simulink model "frenagem_real"  (R2016a)
settings: Solver=ode45  StartTime=0.0  StopTime=200  FixedStep=.03  MaxStep=.1  RelTol=1e-3
libraries: canmsglib x4
settings Model: Creator=vmaraccini  LastModifiedBy=vmaraccini-personal
settings DataIOCC: LimitDataPoints=on  SaveFormat=Array
settings HardwareCC: ProdBitPerPointer=32  ProdLargestAtomicFloat=None  ProdIntDivRoundTo=Undefined  ProdEndianess=Unspecified  ProdWordSize=32  ProdHWDeviceType=32-bit Generic
settings ModelReferenceCC: PropagateSignalLabelsOutOfModel=off
settings ConfigComp: CovModelRefEnable=Off

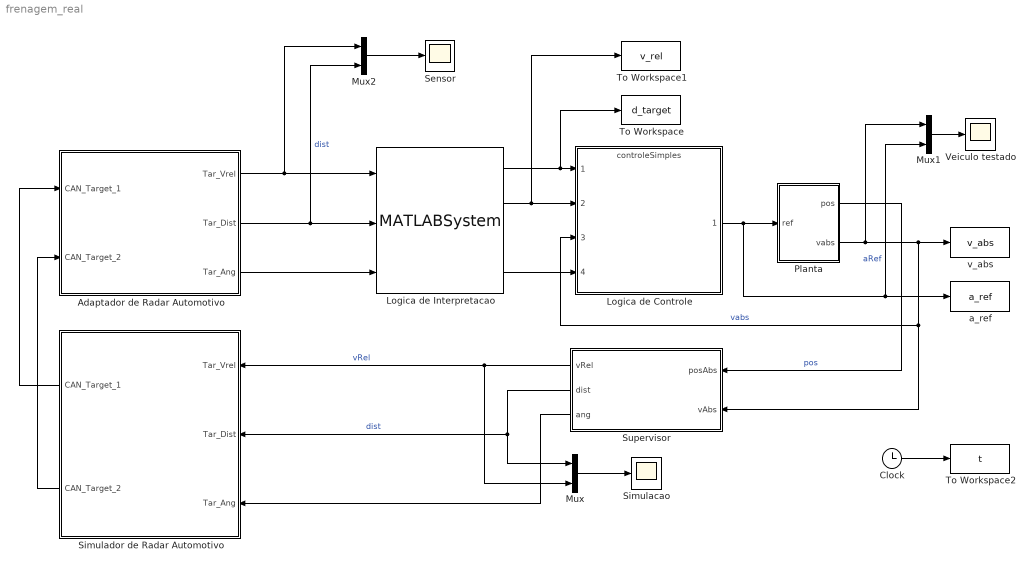
== system frenagem_real ==
  Adaptador de Radar Automotivo : Subsystem
  Clock : Clock
  Logica de Controle : ModelReference  ModelNameDialog=controleSimples.slx  SimulationMode=Normal  ModelReferenceVersion=1.103
  Logica de Interpretacao : MATLABSystem  System=Interpretacao  SimulateUsing=Interpreted execution
      mask Type: Interpretacao
      mask Display:
      | disp('Interpretacao');
      | port_label('input',1,'vrels');
      | port_label('input',2,'dists');
      | port_label('input',3,'angs');
      | port_label('output',1,'dist');
      | port_label('output',2,'vrel');
      | port_label('output',3,'ang');
      | port_label('output',4,'vmax');
  Mux : Mux  Inputs=2
  Mux1 : Mux  Inputs=2
  Mux2 : Mux  Inputs=2
  Planta : Subsystem
  Sensor : Scope
  Simulacao : Scope
  Simulador de Radar Automotivo : Subsystem
  Supervisor : Subsystem
  To Workspace : ToWorkspace  VariableName=d_target  SampleTime=-1
      settings: Save2DSignal=2-D array (concatenate along first dimension)
  To Workspace1 : ToWorkspace  VariableName=v_rel  SampleTime=-1
      settings: Save2DSignal=2-D array (concatenate along first dimension)
  To Workspace2 : ToWorkspace  VariableName=t  SampleTime=-1
      settings: Save2DSignal=2-D array (concatenate along first dimension)
  Veiculo testado : Scope
  a_ref : ToWorkspace  VariableName=a_ref  SampleTime=-1
      settings: Save2DSignal=2-D array (concatenate along first dimension)
  v_abs : ToWorkspace  VariableName=v_abs  SampleTime=-1
      settings: Save2DSignal=2-D array (concatenate along first dimension)
  wires:
  Planta/2(vabs) -> Supervisor/2(vAbs), Logica de Controle/3, v_abs/1, Mux1/1  "vabs"
  Logica de Controle/1 -> Planta/1(ref), Mux1/2, a_ref/1  "aRef"
  Planta/1(pos) -> Supervisor/1(posAbs)  "pos"
  Simulador de Radar Automotivo/1(CAN_Target_1) -> Adaptador de Radar Automotivo/1(CAN_Target_1)
  Simulador de Radar Automotivo/2(CAN_Target_2) -> Adaptador de Radar Automotivo/2(CAN_Target_2)
  Logica de Interpretacao/1 -> To Workspace/1, Logica de Controle/1
  Supervisor/1(vRel) -> Simulador de Radar Automotivo/1(Tar_Vrel), Mux/2  "vRel"
  Supervisor/2(dist) -> Simulador de Radar Automotivo/2(Tar_Dist), Mux/1  "dist"
  Mux/1 -> Simulacao/1
  Mux1/1 -> Veiculo testado/1
  Logica de Interpretacao/4 -> Logica de Controle/4
  Logica de Interpretacao/2 -> Logica de Controle/2, To Workspace1/1
  Supervisor/3(ang) -> Simulador de Radar Automotivo/3(Tar_Ang)
  Adaptador de Radar Automotivo/3(Tar_Ang) -> Logica de Interpretacao/3
  Adaptador de Radar Automotivo/1(Tar_Vrel) -> Mux2/1, Logica de Interpretacao/1
  Adaptador de Radar Automotivo/2(Tar_Dist) -> Mux2/2, Logica de Interpretacao/2  "dist"
  Mux2/1 -> Sensor/1
  Clock/1 -> To Workspace2/1

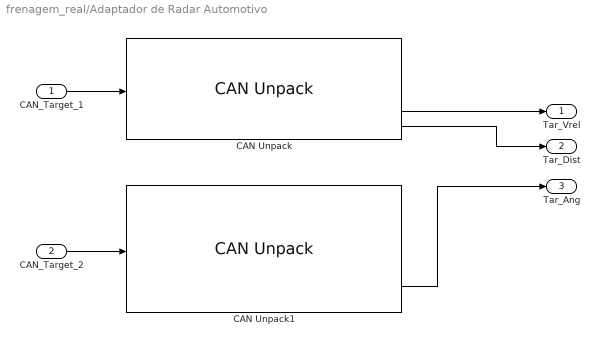
== system frenagem_real/Adaptador de Radar Automotivo ==
  CAN_Target_1 : Inport
  CAN_Target_2 : Inport  Port=2
  CAN Unpack : canmsglib/CAN Unpack  MsgList=(none)  MsgName=CAN1_Target_1  MsgIDType=Standard (11-bit identifier)  MsgIdentifier=1793  MsgLength=8  SignalInfo=NoOfTarget_1$0$8$2$2$1$0$1$0$-Inf$Inf$#Tar_Dist_rms$8$8$2$2$1$0$0.1$-10$-Inf$Inf$#Tar_Ang_rms$17$7$2$2$1$0$0.1$0$-Inf$Inf$#Tar_Vrel_rms$24$9$2$2$1$0$0.03$-5$-Inf$Inf$#Tar_Vrel$44$12$2$2$1$0$0.03$-25$-Inf$Inf$#Tar_Dist$48$11$2$1$1$0$0.1$0$-Inf$Inf$#  NSignals=6  IDPort=off  TimestampPort=off  ErrorPort=off  RemotePort=off  LengthPort=off  StatusPort=off  StartBits=str2num('[int32(0);int32(8);int32(17);int32(24);int32(44);int32(48)]')  SignalSizes=str2num('[int32(8);int32(8);int32(7);int32(9);int32(12);int32(11)]')  ByteOrders=str2num('[int32(2);int32(2);int32(2);int32(2);int32(2);int32(2)]')  DataTypes=str2num('[int32(2);int32(2);int32(2);int32(2);int32(2);int32(1)]')  MultiplexTypes=str2num('[int32(1);int32(1);int32(1);int32(1);int32(1);int32(1)]')  MultiplexValues=str2num('[double(0);double(0);double(0);double(0);double(0);double(0)]')  Factors=str2num('[double(1);double(0.1);double(0.1);double(0.03);double(0.03);double(0.1)]')  Offsets=str2num('[double(0);double(-10);double(0);double(-5);double(-25);double(0)]')  Minimums=str2num('[double(-Inf);double(-Inf);double(-Inf);double(-Inf);double(-Inf);double(-Inf)]')  Maximums=str2num('[double(Inf);double(Inf);double(Inf);double(Inf);double(Inf);double(Inf)]')
  CAN Unpack1 : canmsglib/CAN Unpack  MsgList=(none)  MsgName=CAN1_Target_2  MsgIDType=Standard (11-bit identifier)  MsgIdentifier=1794  MsgLength=8  SignalInfo=NoOfTarget_2$0$8$2$2$1$0$1$0$-Inf$Inf$#Tar_PdH0$9$7$2$2$1$0$0.01$0$-Inf$Inf$#Tar_Length$16$9$2$2$1$0$0.1$0$-Inf$Inf$#Tar_Width$32$9$2$2$1$0$0.1$0$-Inf$Inf$#Tar_Ang_stat$44$2$2$2$1$0$1$0$-Inf$Inf$#Tar_Type$46$2$2$2$1$0$1$0$-Inf$Inf$#Tar_Ang$50$10$2$2$1$0$0.1$-30$-Inf$Inf$#Tar_RCSValue$56$10$2$2$1$0$0.1$-50$-Inf$Inf$#  NSignals=8  IDPort=off  TimestampPort=off  ErrorPort=off  RemotePort=off  LengthPort=off  StatusPort=off  StartBits=str2num('[int32(0);int32(9);int32(16);int32(32);int32(44);int32(46);int32(50);int32(56)]')  SignalSizes=str2num('[int32(8);int32(7);int32(9);int32(9);int32(2);int32(2);int32(10);int32(10)]')  ByteOrders=str2num('[int32(2);int32(2);int32(2);int32(2);int32(2);int32(2);int32(2);int32(2)]')  DataTypes=str2num('[int32(2);int32(2);int32(2);int32(2);int32(2);int32(2);int32(2);int32(2)]')  MultiplexTypes=str2num('[int32(1);int32(1);int32(1);int32(1);int32(1);int32(1);int32(1);int32(1)]')  MultiplexValues=str2num('[double(0);double(0);double(0);double(0);double(0);double(0);double(0);double(0)]')  Factors=str2num('[double(1);double(0.01);double(0.1);double(0.1);double(1);double(1);double(0.1);double(0.1)]')  Offsets=str2num('[double(0);double(0);double(0);double(0);double(0);double(0);double(-30);double(-50)]')  Minimums=str2num('[double(-Inf);double(-Inf);double(-Inf);double(-Inf);double(-Inf);double(-Inf);double(-Inf);double(-Inf)]')  Maximums=str2num('[double(Inf);double(Inf);double(Inf);double(Inf);double(Inf);double(Inf);double(Inf);double(Inf)]')
  Tar_Vrel : Outport
  Tar_Dist : Outport  Port=2
  Tar_Ang : Outport  Port=3
  wires:
  CAN Unpack/6 -> Tar_Dist/1
  CAN Unpack1/7 -> Tar_Ang/1
  CAN Unpack/5 -> Tar_Vrel/1
  CAN_Target_2/1 -> CAN Unpack1/1
  CAN_Target_1/1 -> CAN Unpack/1

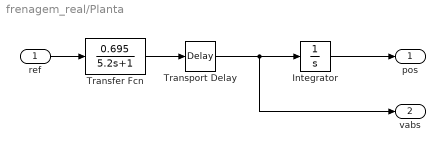
== system frenagem_real/Planta ==
  ref : Inport
  Integrator : Integrator
  Transfer Fcn : TransferFcn  Numerator=[0 0.695]  Denominator=[5.2 1]
  Transport Delay : TransportDelay  DelayTime=0.5
  pos : Outport
  vabs : Outport  Port=2
  wires:
  Integrator/1 -> pos/1
  Transfer Fcn/1 -> Transport Delay/1
  ref/1 -> Transfer Fcn/1
  Transport Delay/1 -> vabs/1, Integrator/1

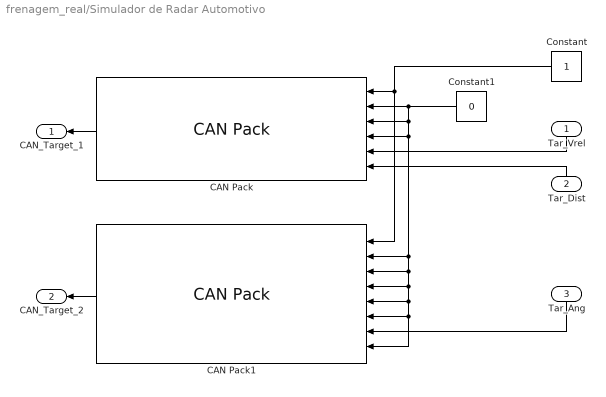
== system frenagem_real/Simulador de Radar Automotivo ==
  Tar_Vrel : Inport
  Tar_Dist : Inport  Port=2
  Tar_Ang : Inport  Port=3
  CAN Pack : canmsglib/CAN Pack  MsgList=(none)  MsgName=CAN1_Target_1  MsgIDType=Standard (11-bit identifier)  MsgIdentifier=1793  MsgLength=8  SignalInfo=NoOfTarget_1$0$8$2$2$1$0$1$0$-Inf$Inf$#Tar_Dist_rms$8$8$2$2$1$0$0.1$-10$-Inf$Inf$#Tar_Ang_rms$17$7$2$2$1$0$0.1$0$-Inf$Inf$#Tar_Vrel_rms$24$9$2$2$1$0$0.03$-5$-Inf$Inf$#Tar_Vrel$44$12$2$2$1$0$0.03$-25$-Inf$Inf$#Tar_Dist$48$11$2$2$1$0$0.1$0$-Inf$Inf$#  NSignals=6  StartBits=str2num('[int32(0);int32(8);int32(17);int32(24);int32(44);int32(48)]')  SignalSizes=str2num('[int32(8);int32(8);int32(7);int32(9);int32(12);int32(11)]')  ByteOrders=str2num('[int32(2);int32(2);int32(2);int32(2);int32(2);int32(2)]')  DataTypes=str2num('[int32(2);int32(2);int32(2);int32(2);int32(2);int32(2)]')  MultiplexTypes=str2num('[int32(1);int32(1);int32(1);int32(1);int32(1);int32(1)]')  MultiplexValues=str2num('[double(0);double(0);double(0);double(0);double(0);double(0)]')  Factors=str2num('[double(1);double(0.1);double(0.1);double(0.03);double(0.03);double(0.1)]')  Offsets=str2num('[double(0);double(-10);double(0);double(-5);double(-25);double(0)]')  Minimums=str2num('[double(-Inf);double(-Inf);double(-Inf);double(-Inf);double(-Inf);double(-Inf)]')  Maximums=str2num('[double(Inf);double(Inf);double(Inf);double(Inf);double(Inf);double(Inf)]')  Remote=off
      settings: DataFormat=manually specified signals
  CAN Pack1 : canmsglib/CAN Pack  MsgList=(none)  MsgName=CAN1_Target_2  MsgIDType=Standard (11-bit identifier)  MsgIdentifier=1794  MsgLength=8  SignalInfo=NoOfTarget_2$0$8$2$2$1$0$1$0$-Inf$Inf$#Tar_PdH0$9$7$2$2$1$0$0.01$-10$-Inf$Inf$#Tar_Length$16$9$2$2$1$0$0.1$0$-Inf$Inf$#Tar_Width$32$9$2$2$1$0$.01$0$-Inf$Inf$#Tar_Ang_stat$44$2$2$2$1$0$1$0$-Inf$Inf$#Tar_Type$46$2$2$2$1$0$1$0$-Inf$Inf$#Tar_Ang$50$10$2$2$1$0$0.1$-30$-Inf$Inf$#Tar_RCSValue$56$10$2$2$1$0$0.1$-50$-Inf$Inf$#  NSignals=8  StartBits=str2num('[int32(0);int32(9);int32(16);int32(32);int32(44);int32(46);int32(50);int32(56)]')  SignalSizes=str2num('[int32(8);int32(7);int32(9);int32(9);int32(2);int32(2);int32(10);int32(10)]')  ByteOrders=str2num('[int32(2);int32(2);int32(2);int32(2);int32(2);int32(2);int32(2);int32(2)]')  DataTypes=str2num('[int32(2);int32(2);int32(2);int32(2);int32(2);int32(2);int32(2);int32(2)]')  MultiplexTypes=str2num('[int32(1);int32(1);int32(1);int32(1);int32(1);int32(1);int32(1);int32(1)]')  MultiplexValues=str2num('[double(0);double(0);double(0);double(0);double(0);double(0);double(0);double(0)]')  Factors=str2num('[double(1);double(0.01);double(0.1);double(.01);double(1);double(1);double(0.1);double(0.1)]')  Offsets=str2num('[double(0);double(-10);double(0);double(0);double(0);double(0);double(-30);double(-50)]')  Minimums=str2num('[double(-Inf);double(-Inf);double(-Inf);double(-Inf);double(-Inf);double(-Inf);double(-Inf);double(-Inf)]')  Maximums=str2num('[double(Inf);double(Inf);double(Inf);double(Inf);double(Inf);double(Inf);double(Inf);double(Inf)]')  Remote=off
      settings: DataFormat=manually specified signals
  Constant : Constant
  Constant1 : Constant  Value=0
  CAN_Target_1 : Outport
  CAN_Target_2 : Outport  Port=2
  wires:
  CAN Pack/1 -> CAN_Target_1/1
  CAN Pack1/1 -> CAN_Target_2/1
  Constant/1 -> CAN Pack1/1, CAN Pack/1
  Tar_Ang/1 -> CAN Pack1/7
  Constant1/1 -> CAN Pack1/8, CAN Pack1/6, CAN Pack1/5, CAN Pack1/4, CAN Pack1/3, CAN Pack1/2, CAN Pack/4, CAN Pack/3, CAN Pack/2
  Tar_Dist/1 -> CAN Pack/6
  Tar_Vrel/1 -> CAN Pack/5

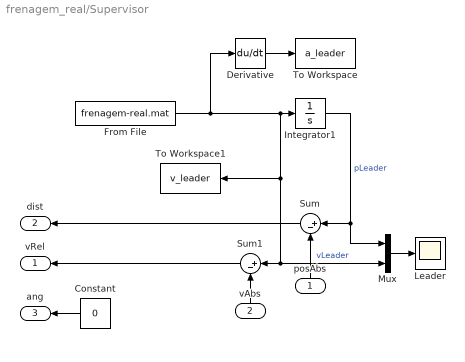
== system frenagem_real/Supervisor ==
  posAbs : Inport
  vAbs : Inport  Port=2
  Constant : Constant  Value=0
  Derivative : Derivative
  From File : FromFile  FileName=frenagem-real.mat  SampleTime=0
  Integrator1 : Integrator  InitialCondition=40
  Leader : Scope
  Mux : Mux  Inputs=2
  Sum : Sum  Inputs=|+-
  Sum1 : Sum  Inputs=|+-
  To Workspace : ToWorkspace  VariableName=a_leader  SampleTime=-1
      settings: Save2DSignal=2-D array (concatenate along first dimension)
  To Workspace1 : ToWorkspace  VariableName=v_leader  SampleTime=-1
      settings: Save2DSignal=2-D array (concatenate along first dimension)
  vRel : Outport
  dist : Outport  Port=2
  ang : Outport  Port=3
  wires:
  Integrator1/1 -> Mux/1, Sum/1  "pLeader"
  Sum1/1 -> vRel/1
  vAbs/1 -> Sum1/2
  posAbs/1 -> Sum/2
  Sum/1 -> dist/1
  From File/1 -> Derivative/1, To Workspace1/1, Mux/2, Sum1/1, Integrator1/1  "vLeader"
  Constant/1 -> ang/1
  Derivative/1 -> To Workspace/1
  Mux/1 -> Leader/1
